simulink model "test_on_struct"  (R2019b)
settings: Solver=VariableStepAuto  StartTime=0.0  StopTime=inf  RelTol=1e-3
settings Model: DataDictionary=test_on_structure.sldd  Creator=lenovo  LastModifiedBy=lenovo

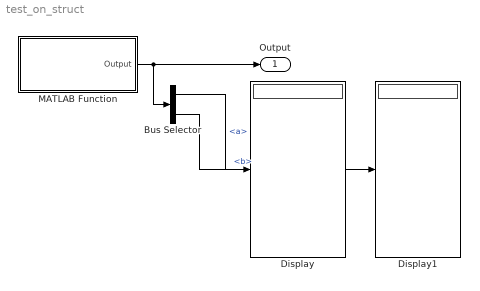
== system test_on_struct ==
  Bus Selector : BusSelector  OutputSignals=a,b
  Display : Display
  Display1 : Display
  MATLAB Function : MATLAB Function  TreatAsAtomicUnit=on
  Output : Outport  OutDataTypeStr=Bus: struct
  wires:
  MATLAB Function/1(Output) -> Bus Selector/1, Output/1
  Bus Selector/1 -> Display/1  "<a>"
  Bus Selector/2 -> Display1/1  "<b>"

== matlab function test_on_struct/MATLAB Function ==
  data: Output output Bus: struct
function Output = fcn()
    y = ones(500,2);
    Output = transition_to_BUS(y);

% y = [1,2,3;4,5,6]';
% Output.a = y(:,1);
% Output.b = y(:,2);

end
    
function Output = transition_to_BUS(output)
    
    if isempty(output)
        output = zeros(500,2);
    else
        size_of_out = length(output);
        if size_of_out <= 500
            output = [output; zeros((500 - size_of_out),2)];
        else
            output = output(1:500,:);
        end
    end
    
    output = randn(500,2);
    Output.a = output(:,1);
    Output.b = output(:,2);
% 
%     Output.a = zeros(3,1);
%     Output.b = zeros(3,1);   
end
